simulink model "yaw_model"  (R2017a)
settings: Solver=ode45  StartTime=0.0  StopTime=200  RelTol=1e-3  EnableMultiTasking=on
values from neighbouring files (symbols this model uses):
  B = 2.8645e-05    [parameters.m]
  Bz = 1.8645e-05    [parameters.m]
  I = Irt+Iw    (= 0.000113883308987)    [parameters.m]
  Iz = IC+I+2*J    (= 0.000744080808987)    [parameters.m]
  Ki_current = 10    [currentController.m]
  KM = 0.075    [parameters.m]
  Kp_current = 13.961    [currentController.m]
  Kv = 0.012    [parameters.m]
  L = (5e-4)*2    (= 0.001)    [parameters.m]
  R = 2*Rfn    (= 3.8)    [parameters.m]
  rad2rpm = 60/(2*pi)    (= 9.54929658551)    [parameters.m]
settings Model: Creator=root  LastModifiedBy=hernan
settings DataIOCC: LimitDataPoints=on  SaveFormat=Array  SignalLoggingSaveFormat=ModelDataLogs
settings OptimizationCC: ExpressionDepthLimit=2147483647  LifeSpan=inf
settings DebuggingCC: UnderspecifiedInitializationDetection=Classic  MergeDetectMultiDrivingBlocksExec=none  SolverPrmCheckMsg=warning  FcnCallInpInsideContextMsg=warning  StateNameClashWarn=warning  SFUnexpectedBacktrackingDiag=warning  SFNoUnconditionalDefaultTransitionDiag=warning  SFExecutionAtInitializationDiag=none
settings HardwareCC: ProdBitPerPointer=32  ProdBitPerSizeT=32  ProdBitPerPtrDiffT=32  ProdLargestAtomicFloat=None  ProdIntDivRoundTo=Undefined  ProdEndianess=Unspecified  ProdWordSize=32  ProdHWDeviceType=32-bit Generic
settings ModelReferenceCC: PropagateSignalLabelsOutOfModel=off
settings GRTTargetCC: TargetLangStandard=C89/C90 (ANSI)  GeneratePreprocessorConditionals=Disable all
settings ConfigComp: CovMetricSettings=dw  CovHtmlReporting=on  CovSaveCumulativeToWorkspaceVar=on  CovSaveSingleToWorkspaceVar=on  CovExternalEMLEnable=off

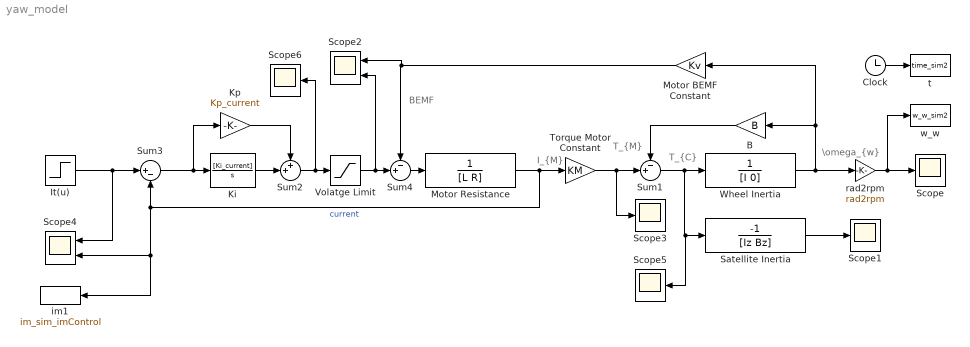
== system yaw_model ==
  note: T_{M}
  note: I_{M}
  note: BEMF
  note: \omega_{w}
  note: T_{C}
  B : Gain  Gain=B
  Clock : Clock
  It(u) : Step  Time=2  After=0.3  SampleTime=0
  Ki : TransferFcn  Numerator=[Ki_current]  Denominator=[1 0]
  Kp : Gain  Gain=Kp_current
  Motor BEMF Constant : Gain  Gain=Kv
  Motor Resistance : TransferFcn  Denominator=[L R]
  Satellite Inertia : TransferFcn  Numerator=[-1]  Denominator=[Iz Bz]
  Scope{,1,3,5..6} (5 alike) : Scope
  Scope2 : Scope  NumInputPorts=2
  Scope4 : Scope  NumInputPorts=2
  Sum1 : Sum  Inputs=-+|
  Sum2 : Sum  Inputs=++|
  Sum3 : Sum  Inputs=|+-
  Sum4 : Sum  Inputs=-+|
  Torque Motor Constant : Gain  Gain=KM
  Volatge Limit : Saturate  UpperLimit=11  LowerLimit=0
  Wheel Inertia : TransferFcn  Denominator=[I 0]
  im1 : ToWorkspace  VariableName=im_sim_imControl  SampleTime=-1
      settings: Save2DSignal=2-D array (concatenate along first dimension)
  rad2rpm : Gain  Gain=rad2rpm
  t : ToWorkspace  VariableName=time_sim2  SampleTime=-1
      settings: Save2DSignal=2-D array (concatenate along first dimension)
  w_w : ToWorkspace  VariableName=w_w_sim2  SampleTime=-1
      settings: Save2DSignal=2-D array (concatenate along first dimension)
  wires:
  Sum4/1 -> Motor Resistance/1
  Torque Motor Constant/1 -> Sum1/2, Scope3/1
  Motor BEMF Constant/1 -> Scope2/1, Sum4/1
  Wheel Inertia/1 -> rad2rpm/1, Motor BEMF Constant/1, B/1
  rad2rpm/1 -> w_w/1, Scope/1
  Clock/1 -> t/1
  Sum1/1 -> Scope5/1, Satellite Inertia/1, Wheel Inertia/1
  B/1 -> Sum1/1
  Satellite Inertia/1 -> Scope1/1
  Sum2/1 -> Volatge Limit/1, Scope6/1
  Kp/1 -> Sum2/1
  Ki/1 -> Sum2/2
  Motor Resistance/1 -> Torque Motor Constant/1, im1/1, Scope4/2, Sum3/2  "current"
  Sum3/1 -> Kp/1, Ki/1
  It(u)/1 -> Scope4/1, Sum3/1
  Volatge Limit/1 -> Scope2/2, Sum4/2
